simulink model "main"  (R2022a)
settings: Solver=FixedStepDiscrete  StartTime=0.0  StopTime=Inf  FixedStep=(50e-6)-(sim_en*4.995e-5)  RelTol=1e-3  EnableMultiTasking=on
model workspace (MAT data in the model file):
  Param : Simulink.Parameter (value not decoded)
  ac_ok : Simulink.Signal (value not decoded)
  ac_ok_120 : Simulink.Signal (value not decoded)
  bulk_voltage : Simulink.Signal (value not decoded)
  burstduty_integ_max : Simulink.Signal (value not decoded)
  burstduty_integ_min : Simulink.Signal (value not decoded)
  burstduty_ki : Simulink.Signal (value not decoded)
  burstduty_kp : Simulink.Signal (value not decoded)
  calib_ok : Simulink.Signal (value not decoded)
  can_addr1 : Simulink.Signal (value not decoded)
  can_addr2 : Simulink.Signal (value not decoded)
  can_addr3 : Simulink.Signal (value not decoded)
  can_addr4 : Simulink.Signal (value not decoded)
  can_data_rx : Simulink.Signal (value not decoded)
  can_data_tx : Simulink.Signal (value not decoded)
  can_timeout_120 : Simulink.Signal (value not decoded)
  chksum_scircv : Simulink.Signal (value not decoded)
  clllc_en_120 : Simulink.Signal (value not decoded)
  clllc_fault_120 : Simulink.Signal (value not decoded)
  clllc_ok_120 : Simulink.Signal (value not decoded)
  cmpss1h : Simulink.Signal (value not decoded)
  cmpss1l : Simulink.Signal (value not decoded)
  cmpss2h : Simulink.Signal (value not decoded)
  cmpss2l : Simulink.Signal (value not decoded)
  cmpss3h : Simulink.Signal (value not decoded)
  cmpss3l : Simulink.Signal (value not decoded)
  cmpss4h : Simulink.Signal (value not decoded)
  cmpss4l : Simulink.Signal (value not decoded)
  cmpss5h : Simulink.Signal (value not decoded)
  cmpss5l : Simulink.Signal (value not decoded)
  cmpss6h : Simulink.Signal (value not decoded)
  cmpss6l : Simulink.Signal (value not decoded)
  cmpss7h : Simulink.Signal (value not decoded)
  cmpss7l : Simulink.Signal (value not decoded)
  cmpss8h : Simulink.Signal (value not decoded)
  cmpss8l : Simulink.Signal (value not decoded)
  cnt_idle : Simulink.Signal (value not decoded)
  cnt_orps : Simulink.Signal (value not decoded)
  cnt_scircv : Simulink.Signal (value not decoded)
  cnt_scixmt : Simulink.Signal (value not decoded)
  cnt_scixmt_func : Simulink.Signal (value not decoded)
  cnt_temp_mux : Simulink.Signal (value not decoded)
  cnt_vdroop : Simulink.Signal (value not decoded)
  config_ok : Simulink.Signal (value not decoded)
  control_en : Simulink.Signal (value not decoded)
  cp_ready_120 : Simulink.Signal (value not decoded)
  d2d_en : Simulink.Signal (value not decoded)
  dchg_off : Simulink.Signal (value not decoded)
  debug_dacb : Simulink.Signal (value not decoded)
  debug_dacc : Simulink.Signal (value not decoded)
  debug_msg1 : Simulink.Signal (value not decoded)
  debug_msg2 : Simulink.Signal (value not decoded)
  debug_msg3 : Simulink.Signal (value not decoded)
  debug_msg4 : Simulink.Signal (value not decoded)
  debug_msg5 : Simulink.Signal (value not decoded)
  debug_msg6 : Simulink.Signal (value not decoded)
  dir_v2g : Simulink.Signal (value not decoded)
  eoss_llc1 : Simulink.Signal (value not decoded)
  eoss_llc2 : Simulink.Signal (value not decoded)
  eoss_orps : Simulink.Signal (value not decoded)
  fault_ocp : Simulink.Signal (value not decoded)
  fault_otp : Simulink.Signal (value not decoded)
  fault_ovp : Simulink.Signal (value not decoded)
  fut_en : Simulink.Signal (value not decoded)
  fwd_en_120 : Simulink.Signal (value not decoded)
  gain_llc1_sec_idc : Simulink.Signal (value not decoded)
  gain_llc1_temp_sr : Simulink.Signal (value not decoded)
  gain_llc2_sec_idc : Simulink.Signal (value not decoded)
  gain_vbat : Simulink.Signal (value not decoded)
  gain_vbulk : Simulink.Signal (value not decoded)
  gain_vout : Simulink.Signal (value not decoded)
  input_current_phasea : Simulink.Signal (value not decoded)
  input_current_phaseb : Simulink.Signal (value not decoded)
  input_current_phasec : Simulink.Signal (value not decoded)
  input_freq : Simulink.Signal (value not decoded)
  input_power : Simulink.Signal (value not decoded)
  input_voltage_phasea : Simulink.Signal (value not decoded)
  input_voltage_phaseb : Simulink.Signal (value not decoded)
  input_voltage_phasec : Simulink.Signal (value not decoded)
  ishare_arbiter : Simulink.Signal (value not decoded)
  ishare_thresh : Simulink.Signal (value not decoded)
  led_g : Simulink.Signal (value not decoded)
  led_r : Simulink.Signal (value not decoded)
  led_y : Simulink.Signal (value not decoded)
  llc1_burst_integ : Simulink.Signal (value not decoded)
  llc1_burstduty_buffer : Simulink.Signal (value not decoded)
  llc1_pfm_error : Simulink.Signal (value not decoded)
  llc1_pfm_integ : Simulink.Signal (value not decoded)
  llc1_pfm_prop : Simulink.Signal (value not decoded)
  llc1_pri_idc : Simulink.Signal (value not decoded)
  llc1_ps_buffer : Simulink.Signal (value not decoded)
  llc1_pspwm_error : Simulink.Signal (value not decoded)
  llc1_pspwm_integ : Simulink.Signal (value not decoded)
  llc1_pspwm_prop : Simulink.Signal (value not decoded)
  llc1_sec_idc : Simulink.Signal (value not decoded)
  llc1_temp_sr : Simulink.Signal (value not decoded)
  llc1_ts_tbctr_buffer : Simulink.Signal (value not decoded)
  llc2_burst_integ : Simulink.Signal (value not decoded)
  llc2_burstduty_buffer : Simulink.Signal (value not decoded)
  llc2_en : Simulink.Signal (value not decoded)
  llc2_en_buffer : Simulink.Signal (value not decoded)
  llc2_pfm_error : Simulink.Signal (value not decoded)
  llc2_pfm_integ : Simulink.Signal (value not decoded)
  llc2_pfm_prop : Simulink.Signal (value not decoded)
  llc2_pri_idc : Simulink.Signal (value not decoded)
  llc2_ps_buffer : Simulink.Signal (value not decoded)
  llc2_pspwm_error : Simulink.Signal (value not decoded)
  llc2_pspwm_integ : Simulink.Signal (value not decoded)
  llc2_pspwm_prop : Simulink.Signal (value not decoded)
  llc2_sec_idc : Simulink.Signal (value not decoded)
  llc2_temp_sr : Simulink.Signal (value not decoded)
  llc2_ts_tbctr_buffer : Simulink.Signal (value not decoded)
  loop_adcint : Simulink.Signal (value not decoded)
  loop_control : Simulink.Signal (value not decoded)
  loop_idle : Simulink.Signal (value not decoded)
  mid_bulk_voltage : Simulink.Signal (value not decoded)
  mode_120 : Simulink.Signal (value not decoded)
  mode_cc_cv : Simulink.Signal (value not decoded)
  myParam : mpt.Parameter (value not decoded)
  obc_ok_120 : Simulink.Signal (value not decoded)
  offset_llc1_sec_idc : Simulink.Signal (value not decoded)
  offset_llc1_temp_sr : Simulink.Signal (value not decoded)
  offset_llc2_sec_idc : Simulink.Signal (value not decoded)
  offset_vbat : Simulink.Signal (value not decoded)
  offset_vbulk : Simulink.Signal (value not decoded)
  offset_vout : Simulink.Signal (value not decoded)
  openloop_en : Simulink.Signal (value not decoded)
  openloop_fault_en : Simulink.Signal (value not decoded)
  ot_fault_120 : Simulink.Signal (value not decoded)
  pfc_en : Simulink.Signal (value not decoded)
  pfc_en_120 : Simulink.Signal (value not decoded)
  pfc_fw_revision : Simulink.Signal (value not decoded)
  pfc_fw_revision_bootloader : Simulink.Signal (value not decoded)
  pfc_fw_revision_debug : Simulink.Signal (value not decoded)
  pfc_ok : Simulink.Signal (value not decoded)
  pfc_ok_120 : Simulink.Signal (value not decoded)
  pfm_a0 : Simulink.Signal (value not decoded)
  pfm_a1 : Simulink.Signal (value not decoded)
  pfm_integ_max : Simulink.Signal (value not decoded)
  pfm_integ_min : Simulink.Signal (value not decoded)
  pfm_ki : Simulink.Signal (value not decoded)
  pfm_kp : Simulink.Signal (value not decoded)
  pri_fut_en : Simulink.Signal (value not decoded)
  pri_fut_en_buffer : Simulink.Signal (value not decoded)
  pri_halfbridge_en : Simulink.Signal (value not decoded)
  pri_halfbridge_en_buffer : Simulink.Signal (value not decoded)
  pspwm_integ_max : Simulink.Signal (value not decoded)
  pspwm_integ_min : Simulink.Signal (value not decoded)
  pspwm_ki : Simulink.Signal (value not decoded)
  pspwm_kp : Simulink.Signal (value not decoded)
  ref_idclink_max : Simulink.Signal (value not decoded)
  ref_iout : Simulink.Signal (value not decoded)
  ref_iout_calib : Simulink.Signal (value not decoded)
  ref_iout_llc1 : Simulink.Signal (value not decoded)
  ref_iout_llc1_calib : Simulink.Signal (value not decoded)
  ref_iout_llc2 : Simulink.Signal (value not decoded)
  ref_iout_llc2_calib : Simulink.Signal (value not decoded)
  ref_pout : Simulink.Signal (value not decoded)
  ref_ss_llc1 : Simulink.Signal (value not decoded)
  ref_ss_llc2 : Simulink.Signal (value not decoded)
  ref_ss_orps : Simulink.Signal (value not decoded)
  ref_vbat : Simulink.Signal (value not decoded)
  ref_vbat_calib : Simulink.Signal (value not decoded)
  ref_vbulk : Simulink.Signal (value not decoded)
  ref_vbulk_calib : Simulink.Signal (value not decoded)
  ref_vbulk_llc1_calib : Simulink.Signal (value not decoded)
  ref_vbulk_llc2_calib : Simulink.Signal (value not decoded)
  ref_vout : Simulink.Signal (value not decoded)
  ref_vout_calib : Simulink.Signal (value not decoded)
  relay_en : Simulink.Signal (value not decoded)
  reset_flag : Simulink.Signal (value not decoded)
  rev_en_120 : Simulink.Signal (value not decoded)
  runtime_control : Simulink.Signal (value not decoded)
  runtime_idle : Simulink.Signal (value not decoded)
  scircv_buffer : Simulink.Signal (value not decoded)
  scircv_buffer_tmp : Simulink.Signal (value not decoded)
  scircv_buffer_tmp_idx0 : Simulink.Signal (value not decoded)
  scircv_chksum : Simulink.Signal (value not decoded)
  scircv_chksum_ok : Simulink.Signal (value not decoded)
  scircv_parse_ok : Simulink.Signal (value not decoded)
  scixmt_buffer : Simulink.Signal (value not decoded)
  scixmt_chksum : Simulink.Signal (value not decoded)
  scixmt_func : Simulink.Signal (value not decoded)
  scixmt_word0_lsb : Simulink.Signal (value not decoded)
  scixmt_word0_msb : Simulink.Signal (value not decoded)
  scixmt_word1_lsb : Simulink.Signal (value not decoded)
  scixmt_word1_msb : Simulink.Signal (value not decoded)
  scixmt_word2_lsb : Simulink.Signal (value not decoded)
  scixmt_word2_msb : Simulink.Signal (value not decoded)
  scixmt_wr : Simulink.Signal (value not decoded)
  ss_step : Simulink.Signal (value not decoded)
  state_calib : Simulink.Signal (value not decoded)
  state_control : Simulink.Signal (value not decoded)
  state_hkeep : Simulink.Signal (value not decoded)
  status_cmpss : Simulink.Signal (value not decoded)
  status_control : Simulink.Signal (value not decoded)
  status_digin : Simulink.Signal (value not decoded)
  status_digout : Simulink.Signal (value not decoded)
  status_fault : Simulink.Signal (value not decoded)
  status_input : Simulink.Signal (value not decoded)
  status_pfc : Simulink.Signal (value not decoded)
  temp_inlet : Simulink.Signal (value not decoded)
  temp_llc1_fet_hs : Simulink.Signal (value not decoded)
  temp_llc2_fet_hs : Simulink.Signal (value not decoded)
  temp_mux : Simulink.Signal (value not decoded)
  temp_mux_s0 : Simulink.Signal (value not decoded)
  temp_mux_s1 : Simulink.Signal (value not decoded)
  temp_mux_s2 : Simulink.Signal (value not decoded)
  temp_outlet : Simulink.Signal (value not decoded)
  temp_pfc_fet_hsa : Simulink.Signal (value not decoded)
  temp_pfc_fet_hsb : Simulink.Signal (value not decoded)
  temp_pfc_fet_hsc : Simulink.Signal (value not decoded)
  temp_pfc_fet_lsa : Simulink.Signal (value not decoded)
  temp_pfc_fet_lsb : Simulink.Signal (value not decoded)
  temp_pfc_fet_lsc : Simulink.Signal (value not decoded)
  test_mode : Simulink.Signal (value not decoded)
  tfcv_cc : Simulink.Signal (value not decoded)
  tfcv_cc_llc2 : Simulink.Signal (value not decoded)
  tfcv_cv : Simulink.Signal (value not decoded)
  tfcv_sr_en : Simulink.Signal (value not decoded)
  tfv_assert_llc1_pri_idc : Simulink.Signal (value not decoded)
  tfv_assert_llc1_sec_idc : Simulink.Signal (value not decoded)
  tfv_assert_llc1_temp_sr : Simulink.Signal (value not decoded)
  tfv_assert_llc2_pri_idc : Simulink.Signal (value not decoded)
  tfv_assert_llc2_sec_idc : Simulink.Signal (value not decoded)
  tfv_assert_llc2_temp_sr : Simulink.Signal (value not decoded)
  tfv_assert_temp_outlet : Simulink.Signal (value not decoded)
  tfv_assert_vaux_uv : Simulink.Signal (value not decoded)
  tfv_assert_vbat : Simulink.Signal (value not decoded)
  tfv_assert_vbulk : Simulink.Signal (value not decoded)
  tfv_assert_vout : Simulink.Signal (value not decoded)
  tfv_cnt_tz : Simulink.Signal (value not decoded)
  tfv_deassert_llc1_pri_idc : Simulink.Signal (value not decoded)
  tfv_deassert_llc1_sec_idc : Simulink.Signal (value not decoded)
  tfv_deassert_llc1_temp_sr : Simulink.Signal (value not decoded)
  tfv_deassert_llc2_pri_idc : Simulink.Signal (value not decoded)
  tfv_deassert_llc2_sec_idc : Simulink.Signal (value not decoded)
  tfv_deassert_llc2_temp_sr : Simulink.Signal (value not decoded)
  tfv_deassert_temp_outlet : Simulink.Signal (value not decoded)
  tfv_deassert_vaux_uv : Simulink.Signal (value not decoded)
  tfv_deassert_vbat : Simulink.Signal (value not decoded)
  tfv_deassert_vbulk : Simulink.Signal (value not decoded)
  tfv_deassert_vout : Simulink.Signal (value not decoded)
  tfv_llc1_pri_idc : Simulink.Signal (value not decoded)
  tfv_llc1_sec_idc : Simulink.Signal (value not decoded)
  tfv_llc1_temp_sr : Simulink.Signal (value not decoded)
  tfv_llc2_pri_idc : Simulink.Signal (value not decoded)
  tfv_llc2_sec_idc : Simulink.Signal (value not decoded)
  tfv_llc2_temp_sr : Simulink.Signal (value not decoded)
  tfv_temp_outlet : Simulink.Signal (value not decoded)
  tfv_vaux_uv : Simulink.Signal (value not decoded)
  tfv_vbat : Simulink.Signal (value not decoded)
  tfv_vbulk : Simulink.Signal (value not decoded)
  tfv_vout : Simulink.Signal (value not decoded)
  timer_1ms : Simulink.Signal (value not decoded)
  tz : Simulink.Signal (value not decoded)
  valve_en : Simulink.Signal (value not decoded)
  vaux : Simulink.Signal (value not decoded)
  vbat : Simulink.Signal (value not decoded)
  vbulk : Simulink.Signal (value not decoded)
  vout : Simulink.Signal (value not decoded)
undefined symbols (not defined in the file or in its folder): CAN_O_INT, CANA_BASE, Down, GPTRIP1SEL, GPTRIP2SEL, TZ1, TZ2, Up
libraries: hdlsllib x159, simulink x94, c2802xlib x32, c2837xDlib x19, c2807xlib x16, c280xlib x13, canmsglib x8, idelinklib_common x2, c2000lib x1, c281xlib x1
(part 9 of 20)

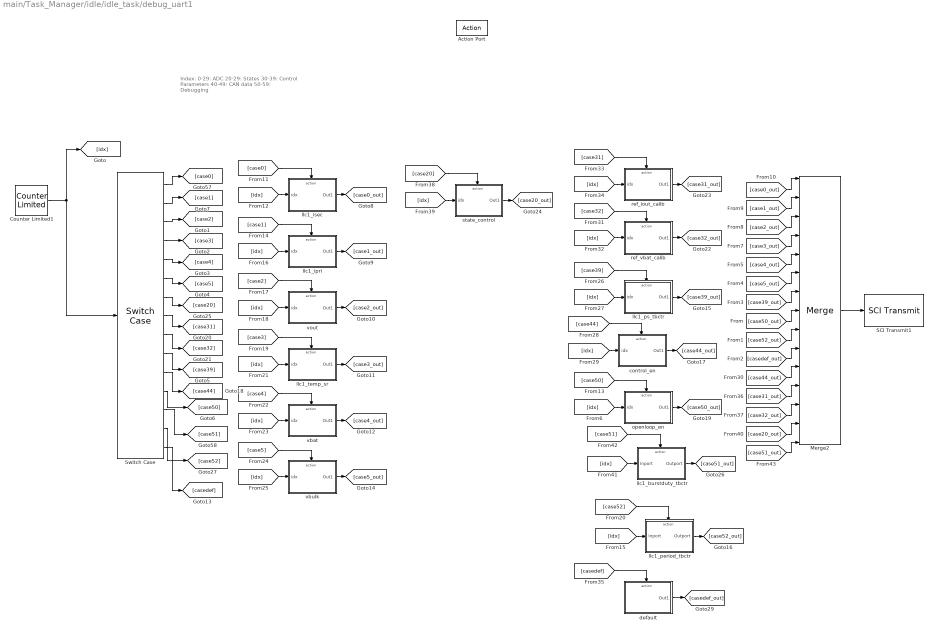
== system main/Task_Manager/idle/idle_task/debug_uart1 ==
  note: Index:
      | 0-29: ADC
      | 20-29: States
      | 30-39: Control Parameters
      | 40-49: CAN data
      | 50-59: Debugging
  Action Port : ActionPort
  Counter Limited1 : simulink/Sources/Counter Limited  uplimit=76  tsamp=-1
  Merge2 : Merge  Inputs=15
  SCI Transmit1 : c280xlib/SCI Transmit  sciModule=A  dataHead='E'  dataTail='S'  blockingMode=on  outputStatus=off
  Switch Case : SwitchCase  CaseConditions={0,1,2,3,4,5,20,31,32,39,44,50,51,52}
  control_en : Subsystem  TreatAsAtomicUnit=on
  default : Subsystem  TreatAsAtomicUnit=on
  llc1_burstduty_tbctr : Subsystem  TreatAsAtomicUnit=on
  llc1_ipri : Subsystem  TreatAsAtomicUnit=on
  llc1_isec : Subsystem  TreatAsAtomicUnit=on
  llc1_period_tbctr : Subsystem  TreatAsAtomicUnit=on
  llc1_ps_tbctr : Subsystem  TreatAsAtomicUnit=on
  llc1_temp_sr : Subsystem  TreatAsAtomicUnit=on
  openloop_en : Subsystem  TreatAsAtomicUnit=on
  ref_iout_calib : Subsystem  TreatAsAtomicUnit=on
  ref_vbat_calib : Subsystem  TreatAsAtomicUnit=on
  state_control : Subsystem  TreatAsAtomicUnit=on
  vbat : Subsystem  TreatAsAtomicUnit=on
  vbulk : Subsystem  TreatAsAtomicUnit=on
  vout : Subsystem  TreatAsAtomicUnit=on
  wires:
  [case51_out] -> Merge2/15
  Switch Case/14 -> [case52]
  [case51] -> llc1_burstduty_tbctr/Action
  [idx] -> llc1_burstduty_tbctr/1(Inport)
  llc1_burstduty_tbctr/1(Outport) -> [case51_out]
  [casedef_out] -> Merge2/10
  [case32_out] -> Merge2/13
  [idx] -> llc1_isec/1(idx)
  [case39_out] -> Merge2/7
  openloop_en/1(Out1) -> [case50_out]
  Merge2/1 -> SCI Transmit1/1
  Counter Limited1/1 -> [idx], Switch Case/1
  [case1_out] -> Merge2/2
  llc1_isec/1(Out1) -> [case0_out]
  Switch Case/10 -> [case39]
  Switch Case/2 -> [case1]
  [idx] -> ref_vbat_calib/1(idx)
  Switch Case/5 -> [case4]
  [idx] -> llc1_ps_tbctr/1(idx)
  default/1(Out1) -> [casedef_out]
  Switch Case/4 -> [case3]
  [case44] -> control_en/Action
  [case39] -> llc1_ps_tbctr/Action
  Switch Case/3 -> [case2]
  [case50_out] -> Merge2/8
  [idx] -> openloop_en/1(idx)
  [casedef] -> default/Action
  [idx] -> vbat/1(idx)
  [case2] -> vout/Action
  llc1_ipri/1(Out1) -> [case1_out]
  llc1_ps_tbctr/1(Out1) -> [case39_out]
  [case3] -> llc1_temp_sr/Action
  [case31_out] -> Merge2/12
  [case0_out] -> Merge2/1
  llc1_period_tbctr/1(Outport) -> [case52_out]
  vout/1(Out1) -> [case2_out]
  [case0] -> llc1_isec/Action
  [idx] -> llc1_temp_sr/1(idx)
  [idx] -> llc1_ipri/1(idx)
  [case4] -> vbat/Action
  [case20_out] -> Merge2/14
  llc1_temp_sr/1(Out1) -> [case3_out]
  [case50] -> openloop_en/Action
  [case2_out] -> Merge2/3
  vbulk/1(Out1) -> [case5_out]
  vbat/1(Out1) -> [case4_out]
  [idx] -> vbulk/1(idx)
  Switch Case/8 -> [case31]
  [idx] -> llc1_period_tbctr/1(Inport)
  [case52_out] -> Merge2/9
  [idx] -> control_en/1(idx)
  [case5] -> vbulk/Action
  Switch Case/6 -> [case5]
  Switch Case/11 -> [case44]
  Switch Case/13 -> [case51]
  [case32] -> ref_vbat_calib/Action
  Switch Case/9 -> [case32]
  [case44_out] -> Merge2/11
  [case5_out] -> Merge2/6
  Switch Case/15 -> [casedef]
  [case3_out] -> Merge2/4
  [case4_out] -> Merge2/5
  [idx] -> ref_iout_calib/1(idx)
  Switch Case/12 -> [case50]
  ref_iout_calib/1(Out1) -> [case31_out]
  [case31] -> ref_iout_calib/Action
  Switch Case/1 -> [case0]
  [idx] -> vout/1(idx)
  [idx] -> state_control/1(idx)
  [case20] -> state_control/Action
  [case1] -> llc1_ipri/Action
  control_en/1(Out1) -> [case44_out]
  [case52] -> llc1_period_tbctr/Action
  ref_vbat_calib/1(Out1) -> [case32_out]
  Switch Case/7 -> [case20]
  state_control/1(Out1) -> [case20_out]

== system main/Task_Manager/idle/idle_task/hkeep ==
  Action Port : ActionPort  ActionPortLabel=case [ 2 ]:
  Function-Call Generator1 : simulink/Ports & Subsystems/Function-Call Generator  sample_time=-1  numberOfIterations=1  DisallowWideOutput=off
  Function-Call Split3 : FunctionCallSplit  NumOutputPorts=2
  tfv : Subsystem  TreatAsAtomicUnit=on
      settings: RTWSystemCode=Inline
  tz : Subsystem  TreatAsAtomicUnit=on
      settings: RTWSystemCode=Inline
  wires:
  Function-Call Split3/1 -> tz/Trigger
  Function-Call Split3/2 -> tfv/Trigger
  Function-Call Generator1/1 -> Function-Call Split3/1

== system main/Task_Manager/idle/idle_task/status ==
  sim_digin : Inport
  Action Port : ActionPort  ActionPortLabel=case [ 3 ]:
  Function-Call Generator : simulink/Ports & Subsystems/Function-Call Generator  sample_time=-1  numberOfIterations=1  DisallowWideOutput=off
  Function-Call Split{,1,3..4} (4 alike) : FunctionCallSplit  NumOutputPorts=2  OutputPortLayout=default
  init : Subsystem  Commented=on  TreatAsAtomicUnit=on
      settings: RTWSystemCode=Inline
  status_control : Subsystem  Commented=on  TreatAsAtomicUnit=on
      settings: RTWSystemCode=Inline
  status_digin : Subsystem  Commented=on  TreatAsAtomicUnit=on
      settings: RTWSystemCode=Inline
  status_digout : Subsystem  Commented=on  TreatAsAtomicUnit=on
      settings: RTWSystemCode=Inline
  status_fault : Subsystem  Commented=on  TreatAsAtomicUnit=on
      settings: RTWSystemCode=Inline
  update_CAN_msg1 : Subsystem  TreatAsAtomicUnit=on
      settings: RTWSystemCode=Inline
  sim_digout : Outport
  wires:
  Function-Call Split3/2 -> status_fault/Trigger
  init/1(sim_digout) -> sim_digout/1
  Function-Call Generator/1 -> Function-Call Split/1
  Function-Call Split3/1 -> Function-Call Split1/1
  Function-Call Split/1 -> Function-Call Split4/1
  sim_digin/1 -> init/1(sim_digin)
  Function-Call Split/2 -> init/Trigger
  Function-Call Split4/2 -> status_control/Trigger
  Function-Call Split4/1 -> Function-Call Split3/1
  Function-Call Split1/2 -> status_digin/Trigger
  Function-Call Split1/1 -> update_CAN_msg1/Trigger

== system main/Task_Manager/idle/idle_task/uartx ==
  Action Port : ActionPort  ActionPortLabel=case [ 4 ]:
  Function-Call Generator1 : simulink/Ports & Subsystems/Function-Call Generator  sample_time=-1  numberOfIterations=1  DisallowWideOutput=off
  Function-Call Split2 : FunctionCallSplit  NumOutputPorts=2
  Function-Call Split4 : FunctionCallSplit  NumOutputPorts=2
  extract_status : Subsystem  TreatAsAtomicUnit=on
  parse : Subsystem  TreatAsAtomicUnit=on
  uart_xmt : Subsystem  TreatAsAtomicUnit=on
  wires:
  Function-Call Split4/1 -> extract_status/Trigger
  Function-Call Split2/1 -> parse/Trigger
  Function-Call Split2/2 -> uart_xmt/Trigger
  Function-Call Split4/2 -> Function-Call Split2/1
  Function-Call Generator1/1 -> Function-Call Split4/1

== system main/Task_Manager/idle/idle_task/watchdog ==
  Action Port : ActionPort  ActionPortLabel=case [ 0 ]:
  Watchdog : c281xlib/Watchdog  resetsrc=Specify via dialog  sample=-1
      settings: SourceProductBaseCode=TIC2000

== system main/Task_Manager/init/codegen/init ==
  Function-Call Generator1 : simulink/Ports & Subsystems/Function-Call Generator  sample_time=-1  numberOfIterations=1  DisallowWideOutput=off
  Function-Call Split{1..3,5} (4 alike) : FunctionCallSplit  NumOutputPorts=2
  cmpss : Subsystem  TreatAsAtomicUnit=on
      settings: RTWSystemCode=Inline
  orps&relay : Subsystem  TreatAsAtomicUnit=on
      settings: RTWSystemCode=Inline
  outputxbar : Subsystem  Commented=on  TreatAsAtomicUnit=on
      settings: RTWSystemCode=Inline
  pwmsync : Subsystem  TreatAsAtomicUnit=on
      settings: RTWSystemCode=Inline
  tztl_clb : Subsystem  Commented=on  TreatAsAtomicUnit=on
      settings: RTWSystemCode=Inline
  wires:
  Function-Call Split5/1 -> cmpss/Trigger
  Function-Call Split5/2 -> Function-Call Split2/1
  Function-Call Split2/1 -> outputxbar/Trigger
  Function-Call Split2/2 -> tztl_clb/Trigger
  Function-Call Split3/2 -> Function-Call Split5/1
  Function-Call Split1/2 -> Function-Call Split3/1
  Function-Call Generator1/1 -> Function-Call Split1/1
  Function-Call Split1/1 -> pwmsync/Trigger
  Function-Call Split3/1 -> orps&relay/Trigger

== system main/interrupt_adca/burst_control/burst/disPulse/Variant Subsystem ==
  note: 1) Add Subsystem or Model blocks as valid variant choices.
      | 2) You cannot connect blocks at this level. At simulation, connectivity is automatically
      | determined, based on the active variant and port name matching.
  dir_v2g : Inport
  codegen : Subsystem  VariantControl=sim_en==0
  sim : Subsystem  VariantControl=sim_en==1

== system main/interrupt_adca/burst_control/burst/disPwm/disPwm ==
  note: 1) Add Subsystem or Model blocks as valid variant choices.
      | 2) You cannot connect blocks at this level. At simulation, connectivity is automatically
      | determined, based on the active variant and port name matching.
  codegen : Subsystem  VariantControl=sim_en==0
  sim : Subsystem  VariantControl=sim_en==1

== system main/interrupt_adca/burst_control/burst/enPulse/enPwm ==
  note: 1) Add Subsystem or Model blocks as valid variant choices.
      | 2) You cannot connect blocks at this level. At simulation, connectivity is automatically
      | determined, based on the active variant and port name matching.
  codegen : Subsystem  VariantControl=sim_en==0
  sim : Subsystem  VariantControl=sim_en==1

== system main/interrupt_adca/get_adc/adc_variant_subsystem/codegen ==
  note: Note:
      | 1. Add ADC debug1 and 2 pending
  note: Note:
      | A0: FWD_CURR_AD  --    J3-30
      | A3: REV_CURR_AD   --    J3-26
      | A5: VO_AD                  --    J7-66
      |
      | B0: AUX_VOLT_AD
      | B3: VBULK_PRI_AD   --  J3- 25
      |
      | D4: T_DD_AD
  sim_adca : Inport
  ADC1 : c2802xlib/ADC  blkParamProc=C2000_Type4  ADCModule=A  samplingMode=Single sample mode  ADCResolution=12-bit (Single-ended input)  useSOC1=SOC0  useSOC2=SOC0_SOC1  SOCAcquisitionWindow=7  SOCTriggerSource=ePWM3_ADCSOCA  SOCInterruptTrigger=No ADCINT  Ts=-1  dType=single  postInterrupt=off  interruptSel=ADCINT1  ADCINTContinuous=on  endma=off  chdma=1  conv1=ADCINA0  conv2=ADCINA0 and ADCINB0  conv1_Type4=ADCIN0  conv2_Type4=ADCIN0 and ADCIN1
  ADC12 : c2802xlib/ADC  blkParamProc=C2000_Type4  ADCModule=D  samplingMode=Single sample mode  ADCResolution=12-bit (Single-ended input)  useSOC1=SOC5  useSOC2=SOC0_SOC1  SOCAcquisitionWindow=7  SOCTriggerSource=Software  SOCInterruptTrigger=No ADCINT  Ts=-1  dType=uint16  postInterrupt=off  interruptSel=ADCINT1  ADCINTContinuous=off  endma=off  chdma=1  conv1=ADCINA0  conv2=ADCINA0 and ADCINB0  conv1_Type4=ADCIN4  conv2_Type4=ADCIN0 and ADCIN1
  ADC2 : c2802xlib/ADC  blkParamProc=C2000_Type4  ADCModule=A  samplingMode=Single sample mode  ADCResolution=12-bit (Single-ended input)  useSOC1=SOC1  useSOC2=SOC0_SOC1  SOCAcquisitionWindow=7  SOCTriggerSource=ePWM3_ADCSOCA  SOCInterruptTrigger=No ADCINT  Ts=-1  dType=single  postInterrupt=off  interruptSel=ADCINT1  ADCINTContinuous=on  endma=off  chdma=1  conv1=ADCINA0  conv2=ADCINA0 and ADCINB0  conv1_Type4=ADCIN3  conv2_Type4=ADCIN0 and ADCIN1
  ADC3 : c2802xlib/ADC  blkParamProc=C2000_Type4  ADCModule=A  samplingMode=Single sample mode  ADCResolution=12-bit (Single-ended input)  useSOC1=SOC2  useSOC2=SOC0_SOC1  SOCAcquisitionWindow=7  SOCTriggerSource=ePWM3_ADCSOCA  SOCInterruptTrigger=No ADCINT  Ts=-1  dType=uint16  postInterrupt=on  interruptSel=ADCINT1  ADCINTContinuous=off  endma=off  chdma=1  conv1=ADCINA0  conv2=ADCINA0 and ADCINB0  conv1_Type4=ADCIN5  conv2_Type4=ADCIN0 and ADCIN1
  ADC6 : c2802xlib/ADC  blkParamProc=C2000_Type4  ADCModule=B  samplingMode=Single sample mode  ADCResolution=12-bit (Single-ended input)  useSOC1=SOC3  useSOC2=SOC0_SOC1  SOCAcquisitionWindow=7  SOCTriggerSource=Software  SOCInterruptTrigger=No ADCINT  Ts=-1  dType=uint16  postInterrupt=off  interruptSel=ADCINT1  ADCINTContinuous=on  endma=off  chdma=1  conv1=ADCINA0  conv2=ADCINA0 and ADCINB0  conv1_Type4=ADCIN0  conv2_Type4=ADCIN0 and ADCIN1
  ADC8 : c2802xlib/ADC  blkParamProc=C2000_Type4  ADCModule=B  samplingMode=Single sample mode  ADCResolution=12-bit (Single-ended input)  useSOC1=SOC4  useSOC2=SOC0_SOC1  SOCAcquisitionWindow=7  SOCTriggerSource=Software  SOCInterruptTrigger=No ADCINT  Ts=-1  dType=uint16  postInterrupt=off  interruptSel=ADCINT1  ADCINTContinuous=off  endma=off  chdma=1  conv1=ADCINA0  conv2=ADCINA0 and ADCINB0  conv1_Type4=ADCIN3  conv2_Type4=ADCIN0 and ADCIN1
  Data Store Write12 : DataStoreWrite  DataStoreName=llc1_sec_idc  IndexOptions=Index vector (dialog)  Indices=1  OutputSizes=1
  Data Store Write17 : DataStoreWrite  DataStoreName=vbat  IndexOptions=Index vector (dialog)  Indices=1  OutputSizes=1
  Data Store Write19 : DataStoreWrite  DataStoreName=vbulk  IndexOptions=Index vector (dialog)  Indices=1  OutputSizes=1
  Data Store Write20 : DataStoreWrite  DataStoreName=vaux  IndexOptions=Index vector (dialog)  Indices=1  OutputSizes=1
  Data Store Write22 : DataStoreWrite  DataStoreName=temp_mux  IndexOptions=Index vector (dialog)  Indices=1  OutputSizes=1
  Data Store Write6 : DataStoreWrite  DataStoreName=llc1_pri_idc  IndexOptions=Index vector (dialog)  Indices=1  OutputSizes=1
  IIR Filter1 : Subsystem
  IIR Filter2 : Subsystem  Commented=on
  IIR Filter3 : Subsystem
  wires:
  ADC3/1 -> Data Store Write17/1
  ADC6/1 -> Data Store Write20/1
  ADC8/1 -> Data Store Write19/1
  ADC12/1 -> Data Store Write22/1
  ADC1/1 -> IIR Filter3/1(x[n])
  ADC2/1 -> IIR Filter1/1(x[n])
  IIR Filter3/1(y[n]) -> Data Store Write12/1
  IIR Filter1/1(y[n]) -> Data Store Write6/1

== system main/interrupt_adca/get_adc/adc_variant_subsystem/sim ==
  sim_adca : Inport
  sim_adcb : Inport  Port=2
  Bus Selector1 : BusSelector  OutputSignals=vbulk,vaux,temp_mux
  Bus Selector2 : BusSelector  OutputSignals=vout,llc1_sec_idc,llc1_pri_idc
  Cast To Single{,1,3..5} (5 alike) : DataTypeConversion  OutDataTypeStr=single  SaturateOnIntegerOverflow=off  RndMeth=Floor
  Data Store Write1 : DataStoreWrite  DataStoreName=llc1_sec_idc  IndexOptions=Index vector (dialog)  Indices=1  OutputSizes=1
  Data Store Write2 : DataStoreWrite  DataStoreName=llc1_pri_idc  IndexOptions=Index vector (dialog)  Indices=1  OutputSizes=1
  Data Store Write23 : DataStoreWrite  DataStoreName=vbulk  IndexOptions=Index vector (dialog)  Indices=1  OutputSizes=1
  Data Store Write25 : DataStoreWrite  DataStoreName=vaux  IndexOptions=Index vector (dialog)  Indices=1  OutputSizes=1
  Data Store Write4 : DataStoreWrite  DataStoreName=vout  IndexOptions=Index vector (dialog)  Indices=1  OutputSizes=1
  Data Store Write6 : DataStoreWrite  DataStoreName=temp_mux  IndexOptions=Index vector (dialog)  Indices=1  OutputSizes=1
  wires:
  [llc1_sec_idc] -> Cast To Single/1
  [llc1_pri_idc] -> Cast To Single1/1
  Bus Selector2/1 -> [vout]  "<vout>"
  Bus Selector2/2 -> [llc1_sec_idc]  "<llc1_sec_idc>"
  Bus Selector2/3 -> [llc1_pri_idc]  "<llc1_pri_idc>"
  sim_adca/1 -> Bus Selector2/1
  sim_adcb/1 -> Bus Selector1/1
  Bus Selector1/1 -> [vbulk]  "<vbulk>"
  Bus Selector1/2 -> [vaux]  "<vaux>"
  [vbulk] -> Cast To Single4/1
  [vaux] -> Cast To Single3/1
  [temp_mux] -> Cast To Single5/1
  Bus Selector1/3 -> [temp_mux]  "<temp_mux>"
  Cast To Single/1 -> Data Store Write1/1
  Cast To Single1/1 -> Data Store Write2/1
  [vout] -> Data Store Write4/1
  Cast To Single3/1 -> Data Store Write25/1
  Cast To Single4/1 -> Data Store Write23/1
  Cast To Single5/1 -> Data Store Write6/1

== system main/interrupt_canrx/canrx_variant_subsystem/codegen/can_rcv ==
  note: Read the CAN Data
  function : TriggerPort  TriggerType=function-call  VariantControl=Variant
  Bitwise AND : simulink/Logic and Bit Operations/Bitwise Operator  logicop=AND  UseBitMask=on  BitMask=hex2dec('0000003F')  BitMaskRealWorld=Stored Integer
  CANA_CAN0INT : idelinklib_common/Memory Copy  Priority=2  copyFrom=Specified source code symbol  copyFromAddressSource=Specify via dialog  copyFromAddress=hex2dec('48108')  copyFromSrcCode=(CANA_BASE + CAN_O_INT)  dataTypeFrom=uint32  dataDimensionFrom=1  useOffsetFrom=off  offsetFromSrc=Specify via dialog  offsetFrom=0  strideFrom=1  copyTo=Output port  copyToAddressSource=Specify via dialog  copyToAddress=hex2dec('00002000')  copyToSrcCode=myVariableDst  dataTypeTo=uint32  useOffsetTo=off  offsetToSrc=Specify via dialog  offsetTo=0  strideTo=1  sampleTime=-1  useInitValue=off  initValueSrc=Specify constant value  initValue=1  initValueSrcCode=myInitValueVariable  useAsMask=off  maskOperator=bitwise AND  useTermValue=off  termValue=1  isRealtimeEnabled=off  emitCCBeforeWrite=off  CCBeforeWrite=/* Custom Code Before Write*/  emitCCAfterWrite=off  CCAfterWrite=/* Custom Code After Write*/  useDMACopy=off  enableBlockingMode=off
      settings: SourceProductBaseCode=ME
  Switch Case : SwitchCase  CaseConditions={10,11,12}  ShowDefaultCase=off
  Switch Case Action Subsystem : Subsystem  TreatAsAtomicUnit=on
  Switch Case Action Subsystem1 : Subsystem  TreatAsAtomicUnit=on
  Switch Case Action Subsystem2 : Subsystem  TreatAsAtomicUnit=on
  wires:
  Switch Case/1 -> Switch Case Action Subsystem/Action
  Switch Case/3 -> Switch Case Action Subsystem2/Action
  Switch Case/2 -> Switch Case Action Subsystem1/Action
  CANA_CAN0INT/1 -> Bitwise AND/1
  Bitwise AND/1 -> Switch Case/1

== system main/Control_State_Machine/control/configSr/configXbarEpwmtrip/codegen/g2v_prifullbridge ==
  Action Port : ActionPort
  Function-Call Generator1 : simulink/Ports & Subsystems/Function-Call Generator  sample_time=-1  numberOfIterations=1  DisallowWideOutput=off
  Function-Call Split3 : FunctionCallSplit  NumOutputPorts=2
  clb : Subsystem  TreatAsAtomicUnit=on
      settings: RTWSystemCode=Inline
  tzctl : Subsystem  TreatAsAtomicUnit=on
      settings: RTWSystemCode=Inline
  wires:
  Function-Call Split3/1 -> tzctl/Trigger
  Function-Call Generator1/1 -> Function-Call Split3/1
  Function-Call Split3/2 -> clb/Trigger

== system main/Control_State_Machine/control/configSr/configXbarEpwmtrip/codegen/v2g_prifullbridge ==
  Action Port : ActionPort
  Function-Call Generator2 : simulink/Ports & Subsystems/Function-Call Generator  sample_time=-1  numberOfIterations=1  DisallowWideOutput=off
  Function-Call Split1 : FunctionCallSplit  NumOutputPorts=2
  clb : Subsystem  TreatAsAtomicUnit=on
      settings: RTWSystemCode=Inline
  tzctl : Subsystem  TreatAsAtomicUnit=on
      settings: RTWSystemCode=Inline
  wires:
  Function-Call Generator2/1 -> Function-Call Split1/1
  Function-Call Split1/1 -> tzctl/Trigger
  Function-Call Split1/2 -> clb/Trigger

== system main/Control_State_Machine/control/configSr/configXbarEpwmtrip/sim/g2v_prifullbridge ==
  Action Port : ActionPort
  Constant{,1..3} (4 alike) : Constant  Value=0  OutDataTypeStr=uint16
  Constant{4,9..11} (4 alike) : Constant  OutDataTypeStr=uint16
  Data Store Write1 : DataStoreWrite  DataStoreName=xbar_epwmtrip_llc1_pri_qb_en  IndexOptions=Index vector (dialog)  Indices=1  OutputSizes=1
  Data Store Write10 : DataStoreWrite  DataStoreName=xbar_epwmtrip_llc1_sec_qd_en  IndexOptions=Index vector (dialog)  Indices=1  OutputSizes=1
  Data Store Write2 : DataStoreWrite  DataStoreName=xbar_epwmtrip_llc1_pri_qc_en  IndexOptions=Index vector (dialog)  Indices=1  OutputSizes=1
  Data Store Write3 : DataStoreWrite  DataStoreName=xbar_epwmtrip_llc1_pri_qd_en  IndexOptions=Index vector (dialog)  Indices=1  OutputSizes=1
  Data Store Write4 : DataStoreWrite  DataStoreName=xbar_epwmtrip_llc1_sec_qa_en  IndexOptions=Index vector (dialog)  Indices=1  OutputSizes=1
  Data Store Write6 : DataStoreWrite  DataStoreName=xbar_epwmtrip_llc1_pri_qa_en  IndexOptions=Index vector (dialog)  Indices=1  OutputSizes=1
  Data Store Write8 : DataStoreWrite  DataStoreName=xbar_epwmtrip_llc1_sec_qb_en  IndexOptions=Index vector (dialog)  Indices=1  OutputSizes=1
  Data Store Write9 : DataStoreWrite  DataStoreName=xbar_epwmtrip_llc1_sec_qc_en  IndexOptions=Index vector (dialog)  Indices=1  OutputSizes=1
  wires:
  Constant3/1 -> Data Store Write3/1
  Constant2/1 -> Data Store Write2/1
  Constant1/1 -> Data Store Write1/1
  Constant/1 -> Data Store Write6/1
  Constant4/1 -> Data Store Write4/1
  Constant9/1 -> Data Store Write8/1
  Constant10/1 -> Data Store Write9/1
  Constant11/1 -> Data Store Write10/1

== system main/Control_State_Machine/control/configSr/configXbarEpwmtrip/sim/v2g_prifullbridge ==
  Action Port : ActionPort
  Constant{,1..3} (4 alike) : Constant  Value=0  OutDataTypeStr=uint16
  Constant{4,9..11} (4 alike) : Constant  OutDataTypeStr=uint16
  Data Store Write1 : DataStoreWrite  DataStoreName=xbar_epwmtrip_llc1_pri_qb_en  IndexOptions=Index vector (dialog)  Indices=1  OutputSizes=1
  Data Store Write10 : DataStoreWrite  DataStoreName=xbar_epwmtrip_llc1_sec_qd_en  IndexOptions=Index vector (dialog)  Indices=1  OutputSizes=1
  Data Store Write2 : DataStoreWrite  DataStoreName=xbar_epwmtrip_llc1_pri_qc_en  IndexOptions=Index vector (dialog)  Indices=1  OutputSizes=1
  Data Store Write3 : DataStoreWrite  DataStoreName=xbar_epwmtrip_llc1_pri_qd_en  IndexOptions=Index vector (dialog)  Indices=1  OutputSizes=1
  Data Store Write4 : DataStoreWrite  DataStoreName=xbar_epwmtrip_llc1_sec_qa_en  IndexOptions=Index vector (dialog)  Indices=1  OutputSizes=1
  Data Store Write6 : DataStoreWrite  DataStoreName=xbar_epwmtrip_llc1_pri_qa_en  IndexOptions=Index vector (dialog)  Indices=1  OutputSizes=1
  Data Store Write8 : DataStoreWrite  DataStoreName=xbar_epwmtrip_llc1_sec_qb_en  IndexOptions=Index vector (dialog)  Indices=1  OutputSizes=1
  Data Store Write9 : DataStoreWrite  DataStoreName=xbar_epwmtrip_llc1_sec_qc_en  IndexOptions=Index vector (dialog)  Indices=1  OutputSizes=1
  wires:
  Constant4/1 -> Data Store Write6/1
  Constant11/1 -> Data Store Write3/1
  Constant10/1 -> Data Store Write2/1
  Constant9/1 -> Data Store Write1/1
  Constant1/1 -> Data Store Write8/1
  Constant2/1 -> Data Store Write9/1
  Constant3/1 -> Data Store Write10/1
  Constant/1 -> Data Store Write4/1

== system main/Control_State_Machine/control/disPwm/disPwm/codegen/System Outputs1 ==

== system main/Control_State_Machine/control/enableSR/enPwm/codegen/System Outputs ==

== system main/Task_Manager/Tmr_1mS/codegen/Task_1mS/Counter_1mS ==
  note: Note:
      |  - Worst error of tfv is timer interval (1ms) + twice the execution of supervisory loop
      |  - Effective max count is 65.536 = 2e16*1e-3
  function : TriggerPort  TriggerType=function-call  VariantControl=Variant
  Add : Sum
  Constant : Constant  OutDataTypeStr=uint16
  Data Store Read : DataStoreRead  DataStoreName=timer_1ms  IndexOptions=Index vector (dialog)  Indices=1  OutputSizes=1
  Data Store Write : DataStoreWrite  DataStoreName=timer_1ms  IndexOptions=Index vector (dialog)  Indices=1  OutputSizes=1
  wires:
  Constant/1 -> Add/2
  Add/1 -> Data Store Write/1
  Data Store Read/1 -> Add/1

== system main/Task_Manager/Tmr_1mS/codegen/Task_1mS/GPIO_Handler ==
  function : TriggerPort  TriggerType=function-call  VariantControl=Variant
  Cast{,1..7} (8 alike) : DataTypeConversion  OutDataTypeStr=boolean  SaturateOnIntegerOverflow=off  RndMeth=Floor
  Constant : Constant
  Constant1 : Constant
  Data Store Read1 : DataStoreRead  DataStoreName=pfc_en_120  IndexOptions=Index vector (dialog)  Indices=1  OutputSizes=1
  Data Store Read2 : DataStoreRead  DataStoreName=obc_ok_120  IndexOptions=Index vector (dialog)  Indices=1  OutputSizes=1
  Data Store Read5 : DataStoreRead  DataStoreName=clllc_ok_120  IndexOptions=Index vector (dialog)  Indices=1  OutputSizes=1
  Data Store Write1 : DataStoreWrite  DataStoreName=ac_ok_120  IndexOptions=Index vector (dialog)  Indices=1  OutputSizes=1
  Data Store Write12 : DataStoreWrite  DataStoreName=cp_ready_120  IndexOptions=Index vector (dialog)  Indices=1  OutputSizes=1
  Data Store Write2 : DataStoreWrite  DataStoreName=pfc_ok_120  IndexOptions=Index vector (dialog)  Indices=1  OutputSizes=1
  Data Store Write3 : DataStoreWrite  DataStoreName=clllc_en_120  IndexOptions=Index vector (dialog)  Indices=1  OutputSizes=1
  Digital Input1 : c2837xDlib/Digital Input  GPIO_Number=GPIO56~GPIO63  GPIO_Bit0=off  GPIO_Bit1=off  GPIO_Bit2=off  GPIO_Bit3=off  GPIO_Bit4=on  GPIO_Bit5=off  GPIO_Bit6=off  GPIO_Bit7=off  sampleTime=0.001  dataType=auto  GPIO_Bit0_Qualification=Sync to SYSCLKOUT  GPIO_Bit1_Qualification=Sync to SYSCLKOUT  GPIO_Bit2_Qualification=Sync to SYSCLKOUT  GPIO_Bit3_Qualification=Sync to SYSCLKOUT  GPIO_Bit4_Qualification=Sync to SYSCLKOUT  GPIO_Bit5_Qualification=Sync to SYSCLKOUT  GPIO_Bit6_Qualification=Sync to SYSCLKOUT  GPIO_Bit7_Qualification=Sync to SYSCLKOUT  Qualification_Period=-1
      settings: SourceProductBaseCode=TIC2000
  Digital Input2 : c2837xDlib/Digital Input  GPIO_Number=GPIO56~GPIO63  GPIO_Bit0=off  GPIO_Bit1=off  GPIO_Bit2=off  GPIO_Bit3=on  GPIO_Bit4=off  GPIO_Bit5=off  GPIO_Bit6=off  GPIO_Bit7=off  sampleTime=0.001  dataType=auto  GPIO_Bit0_Qualification=Sync to SYSCLKOUT  GPIO_Bit1_Qualification=Sync to SYSCLKOUT  GPIO_Bit2_Qualification=Sync to SYSCLKOUT  GPIO_Bit3_Qualification=Sync to SYSCLKOUT  GPIO_Bit4_Qualification=Sync to SYSCLKOUT  GPIO_Bit5_Qualification=Sync to SYSCLKOUT  GPIO_Bit6_Qualification=Sync to SYSCLKOUT  GPIO_Bit7_Qualification=Sync to SYSCLKOUT  Qualification_Period=-1
      settings: SourceProductBaseCode=TIC2000
  Digital Input3 : c2837xDlib/Digital Input  GPIO_Number=GPIO56~GPIO63  GPIO_Bit0=off  GPIO_Bit1=on  GPIO_Bit2=off  GPIO_Bit3=off  GPIO_Bit4=off  GPIO_Bit5=off  GPIO_Bit6=off  GPIO_Bit7=off  sampleTime=0.001  dataType=auto  GPIO_Bit0_Qualification=Sync to SYSCLKOUT  GPIO_Bit1_Qualification=Sync to SYSCLKOUT  GPIO_Bit2_Qualification=Sync to SYSCLKOUT  GPIO_Bit3_Qualification=Sync to SYSCLKOUT  GPIO_Bit4_Qualification=Sync to SYSCLKOUT  GPIO_Bit5_Qualification=Sync to SYSCLKOUT  GPIO_Bit6_Qualification=Sync to SYSCLKOUT  GPIO_Bit7_Qualification=Sync to SYSCLKOUT  Qualification_Period=-1
      settings: SourceProductBaseCode=TIC2000
  Digital Input4 : c2837xDlib/Digital Input  GPIO_Number=GPIO56~GPIO63  GPIO_Bit0=off  GPIO_Bit1=off  GPIO_Bit2=on  GPIO_Bit3=off  GPIO_Bit4=off  GPIO_Bit5=off  GPIO_Bit6=off  GPIO_Bit7=off  sampleTime=0.001  dataType=auto  GPIO_Bit0_Qualification=Sync to SYSCLKOUT  GPIO_Bit1_Qualification=Sync to SYSCLKOUT  GPIO_Bit2_Qualification=Sync to SYSCLKOUT  GPIO_Bit3_Qualification=Sync to SYSCLKOUT  GPIO_Bit4_Qualification=Sync to SYSCLKOUT  GPIO_Bit5_Qualification=Sync to SYSCLKOUT  GPIO_Bit6_Qualification=Sync to SYSCLKOUT  GPIO_Bit7_Qualification=Sync to SYSCLKOUT  Qualification_Period=-1
      settings: SourceProductBaseCode=TIC2000
  Digital Output : c2837xDlib/Digital Output  GPIO_Number=GPIO64~GPIO71  GPIO_Bit0=off  GPIO_BIT0_Toggle=off  GPIO_Bit1=off  GPIO_BIT1_Toggle=off  GPIO_Bit2=off  GPIO_BIT2_Toggle=off  GPIO_Bit3=on  GPIO_BIT3_Toggle=off  GPIO_Bit4=off  GPIO_BIT4_Toggle=off  GPIO_Bit5=off  GPIO_BIT5_Toggle=off  GPIO_Bit6=off  GPIO_BIT6_Toggle=off  GPIO_Bit7=off  GPIO_BIT7_Toggle=off
      settings: SourceProductBaseCode=TIC2000
  Digital Output1 : c2837xDlib/Digital Output  GPIO_Number=GPIO64~GPIO71  GPIO_Bit0=off  GPIO_BIT0_Toggle=off  GPIO_Bit1=off  GPIO_BIT1_Toggle=off  GPIO_Bit2=off  GPIO_BIT2_Toggle=off  GPIO_Bit3=off  GPIO_BIT3_Toggle=off  GPIO_Bit4=on  GPIO_BIT4_Toggle=off  GPIO_Bit5=off  GPIO_BIT5_Toggle=off  GPIO_Bit6=off  GPIO_BIT6_Toggle=off  GPIO_Bit7=off  GPIO_BIT7_Toggle=off
      settings: SourceProductBaseCode=TIC2000
  Digital Output2 : c2837xDlib/Digital Output  GPIO_Number=GPIO48~GPIO55  GPIO_Bit0=off  GPIO_BIT0_Toggle=off  GPIO_Bit1=on  GPIO_BIT1_Toggle=off  GPIO_Bit2=off  GPIO_BIT2_Toggle=off  GPIO_Bit3=off  GPIO_BIT3_Toggle=off  GPIO_Bit4=off  GPIO_BIT4_Toggle=off  GPIO_Bit5=off  GPIO_BIT5_Toggle=off  GPIO_Bit6=off  GPIO_BIT6_Toggle=off  GPIO_Bit7=off  GPIO_BIT7_Toggle=off
      settings: SourceProductBaseCode=TIC2000
  Digital Output3 : c2837xDlib/Digital Output  GPIO_Number=GPIO64~GPIO71  GPIO_Bit0=on  GPIO_BIT0_Toggle=off  GPIO_Bit1=off  GPIO_BIT1_Toggle=off  GPIO_Bit2=off  GPIO_BIT2_Toggle=off  GPIO_Bit3=off  GPIO_BIT3_Toggle=off  GPIO_Bit4=off  GPIO_BIT4_Toggle=off  GPIO_Bit5=off  GPIO_BIT5_Toggle=off  GPIO_Bit6=off  GPIO_BIT6_Toggle=off  GPIO_Bit7=off  GPIO_BIT7_Toggle=off
      settings: SourceProductBaseCode=TIC2000
  Update_ACOK : Subsystem
  Update_CLLLCEN : Subsystem
  Update_CPReady : Subsystem
  Update_PFCOK : Subsystem
  wires:
  Cast3/1 -> Update_CLLLCEN/1(Dig_Input)
  Cast/1 -> Update_ACOK/1(Dig_Input)
  Data Store Read5/1 -> Cast5/1
  Cast1/1 -> Update_PFCOK/1(Dig_Input)
  Digital Input4/1 -> Cast3/1  "CLLLC_EN"
  Data Store Read1/1 -> Cast6/1
  Data Store Read2/1 -> Cast4/1
  Update_CLLLCEN/1(Dig_Input_State) -> Data Store Write3/1
  Update_ACOK/1(Dig_Input_State) -> Data Store Write1/1
  Cast2/1 -> Update_CPReady/1(Dig_Input)
  Update_PFCOK/1(Dig_Input_State) -> Data Store Write2/1
  Cast4/1 -> Digital Output2/1
  Cast6/1 -> Digital Output/1
  Cast5/1 -> Digital Output1/1
  Update_CPReady/1(Dig_Input_State) -> Data Store Write12/1
  Cast7/1 -> Digital Output3/1
  Constant1/1 -> Cast7/1
  Digital Input1/1 -> Cast/1  "CP_READY"
  Digital Input2/1 -> Cast1/1  "PFC_OK"
  Digital Input3/1 -> Cast2/1  "CP_READY"

== system main/Task_Manager/Tmr_1s/codegen/Task_1S/addressing_temp_mux ==
  note: Note:
      | 0   dec0: llc1_temp_sr
      | 1   dec2: llc2_temp_sr
      | 2   dec6: temp_outlet
  function : TriggerPort  TriggerType=function-call  VariantControl=Variant
  Data Store Read1 : DataStoreRead  DataStoreName=cnt_temp_mux  IndexOptions=Index vector (dialog)  Indices=1  OutputSizes=1
  If : If  IfExpression=u1 == 0  ElseIfExpressions=u1 == 1, u1 == 2
  cnt_temp_mux0 : Subsystem  TreatAsAtomicUnit=on
  cnt_temp_mux1 : Subsystem  TreatAsAtomicUnit=on
  cnt_temp_mux2 : Subsystem  TreatAsAtomicUnit=on
  wires:
  Data Store Read1/1 -> If/1
  If/1 -> cnt_temp_mux0/Action
  If/2 -> cnt_temp_mux1/Action
  If/3 -> cnt_temp_mux2/Action

== system main/Task_Manager/Tmr_1s/codegen/Task_1S/cnt_temp_mux ==
  function : TriggerPort  TriggerType=function-call  VariantControl=Variant
  Data Store Read : DataStoreRead  DataStoreName=cnt_temp_mux  IndexOptions=Index vector (dialog)  Indices=1  OutputSizes=1
  If : If  IfExpression=u1 < 3
  cnt_temp_mux : Subsystem  TreatAsAtomicUnit=on
  cnt_temp_mux_sat : Subsystem  TreatAsAtomicUnit=on
  wires:
  If/2 -> cnt_temp_mux_sat/Action
  Data Store Read/1 -> If/1
  If/1 -> cnt_temp_mux/Action

== system main/Task_Manager/Tmr_20mS/codegen/Task_20mS/Rx_Handler ==
  function : TriggerPort  TriggerType=function-call  VariantControl=Variant
  Data Store Read : DataStoreRead  DataStoreName=b05_MB10Received  IndexOptions=Index vector (dialog)  Indices=1  OutputSizes=1
  Data Store Read1 : DataStoreRead  DataStoreName=b06_MB11Received  IndexOptions=Index vector (dialog)  Indices=1  OutputSizes=1
  Data Store Read2 : DataStoreRead  DataStoreName=b07_MB12Received  IndexOptions=Index vector (dialog)  Indices=1  OutputSizes=1
  If : If  NumInputs=3  IfExpression=u1 == 1  ElseIfExpressions=u2 ==1, u3==1
  ProcessMB10 : Subsystem  TreatAsAtomicUnit=on
  ProcessMB11 : Subsystem  TreatAsAtomicUnit=on
  ProcessMB12 : Subsystem  TreatAsAtomicUnit=on
  wires:
  If/1 -> ProcessMB10/Action
  If/2 -> ProcessMB11/Action
  If/3 -> ProcessMB12/Action
  Data Store Read/1 -> If/1
  Data Store Read1/1 -> If/2
  Data Store Read2/1 -> If/3

== system main/Task_Manager/Tmr_20mS/codegen/Task_20mS/Tx_Handler ==
  "function " : TriggerPort  TriggerType=function-call  VariantControl=Variant
  Constant4 : Constant  Value=10  OutDataTypeStr=uint16
  Data Store Read : DataStoreRead  DataStoreName=u16TxDelayCount  IndexOptions=Index vector (dialog)  Indices=1  OutputSizes=1
  Data Store Write1 : DataStoreWrite  DataStoreName=u16TxDelayCount  IndexOptions=Index vector (dialog)  Indices=1  OutputSizes=1
  If2 : If  NumInputs=2  IfExpression=u1 == u2
  Increment Stored Integer : simulink/Additional Math & Discrete/Additional Math: Increment - Decrement/Increment Stored Integer
  Run Tx Routine : Subsystem  TreatAsAtomicUnit=on
  wires:
  Data Store Read/1 -> Increment Stored Integer/1
  Increment Stored Integer/1 -> If2/1, Data Store Write1/1
  Constant4/1 -> If2/2
  If2/1 -> Run Tx Routine/Action

== system main/Task_Manager/idle/idle_task/comm_npc/comm_npc/COMM_NPC.calcScircvChksum ==
  scircv_buffer : Inport
  f : TriggerPort  TriggerType=function-call  VariantControl=(inherit)
      settings: CopyFcn=Stateflow.SLINSF.SimulinkMan.removeBlockPreDeleteFcn  PreDeleteFcn=Stateflow.SLINSF.SimulinkMan.unsafePredeleteFcn
  For Iterator Subsystem : Subsystem  TreatAsAtomicUnit=on
  wires:
  scircv_buffer/1 -> For Iterator Subsystem/1(scircv_buffer)

== system main/Task_Manager/idle/idle_task/comm_npc/comm_npc/COMM_NPC.calcScixmtChksum ==
  note: Note:
      | byte0 - header
      | byte1 - w/r
      | byte2 - func
      | byte3, byte4 - word0_lsb, word0_msb
      | byte5, byte6 - word1_lsb, word1_msb
      | byte7, byte8 - word2_lsb, word2_msb
      | byte9 - chksum
      | byte10 - 0x00
      | byte11 - terminator
  f : TriggerPort  TriggerType=function-call  VariantControl=(inherit)
      settings: CopyFcn=Stateflow.SLINSF.SimulinkMan.removeBlockPreDeleteFcn  PreDeleteFcn=Stateflow.SLINSF.SimulinkMan.unsafePredeleteFcn
  Function-Call Generator1 : simulink/Ports & Subsystems/Function-Call Generator  sample_time=-1  numberOfIterations=1  DisallowWideOutput=off
  Function-Call Split3 : FunctionCallSplit  NumOutputPorts=2
  calc_chksum : Subsystem  TreatAsAtomicUnit=on
      settings: RTWSystemCode=Inline
  update_scixmt_buffer : Subsystem  TreatAsAtomicUnit=on
      settings: RTWSystemCode=Inline
  wires:
  Function-Call Split3/2 -> calc_chksum/Trigger
  Function-Call Split3/1 -> update_scixmt_buffer/Trigger
  Function-Call Generator1/1 -> Function-Call Split3/1
